simulink model "PhaseCompartor"  (Simulink 5.0)
settings: Solver=ode45  StartTime=0.0  StopTime=1000  MaxStep=0.01  RelTol=1e-3
settings Model: LastModifiedBy=thh

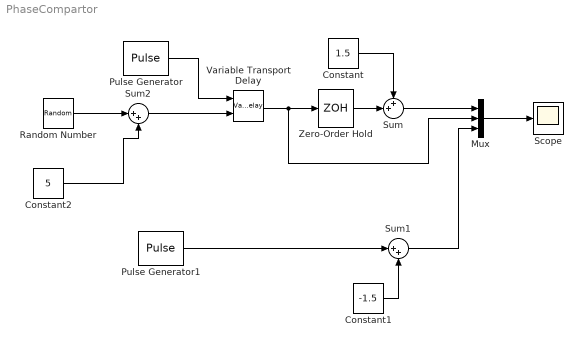
== system PhaseCompartor ==
  Constant : Constant  Value=1.5
  Constant1 : Constant  Value=-1.5
  Constant2 : Constant  Value=5
  Mux : Mux  Inputs=3
  Pulse Generator : DiscretePulseGenerator  PulseType=Time based  Period=11/2*1.01  PulseWidth=50  PhaseDelay=1
  Pulse Generator1 : DiscretePulseGenerator  PulseType=Time based  Period=11  PulseWidth=50
  Random Number : RandomNumber  Variance=0.1  SampleTime=0
  Scope : Scope
      settings: TimeRange=600  YMin=-2  YMax=3
  Sum : Sum  Inputs=++|  SaturateOnIntegerOverflow=on
  Sum1 : Sum  Inputs=|++  SaturateOnIntegerOverflow=on
  Sum2 : Sum  Inputs=|++  SaturateOnIntegerOverflow=on
  Variable Transport Delay : VariableTransportDelay  MaximumDelay=10
  Zero-Order Hold : ZeroOrderHold  SampleTime=11
  wires:
  Mux/1 -> Scope/1
  Sum/1 -> Mux/1
  Zero-Order Hold/1 -> Sum/2
  Constant/1 -> Sum/1
  Sum1/1 -> Mux/3
  Pulse Generator1/1 -> Sum1/1
  Constant1/1 -> Sum1/2
  Variable Transport Delay/1 -> Zero-Order Hold/1, Mux/2
  Pulse Generator/1 -> Variable Transport Delay/1
  Sum2/1 -> Variable Transport Delay/2
  Random Number/1 -> Sum2/1
  Constant2/1 -> Sum2/2
